simulink model "subsystem_converstion"  (R2021a)
settings: Solver=VariableStepAuto  StartTime=0.0  StopTime=10.0  MaxStep=1e-6  RelTol=1e-3
settings Model: Creator=Beshary  LastModifiedBy=Beshary

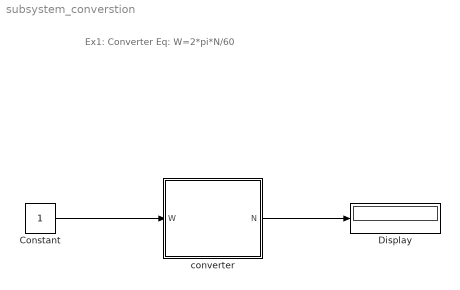
== system subsystem_converstion ==
  note: Ex1: Converter
      | Eq: W=2*pi*N/60
  Constant : Constant
  Display : Display
  converter : Subsystem
  wires:
  Constant/1 -> converter/1(W)
  converter/1(N) -> Display/1

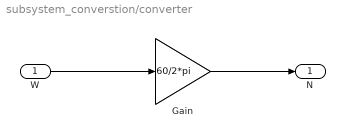
== system subsystem_converstion/converter ==
  W : Inport
  Gain : Gain  Gain=60/2*pi
  N : Outport
  wires:
  Gain/1 -> N/1
  W/1 -> Gain/1
